simulink subsystem "Day1_Scenario_2"  (R2024a)
settings: Solver=VariableStepAuto  StartTime=0.0  StopTime=10.0  RelTol=1e-3
libraries: CarMaker4SL x2
settings Model: Creator=junhyung.cha  LastModifiedBy=User

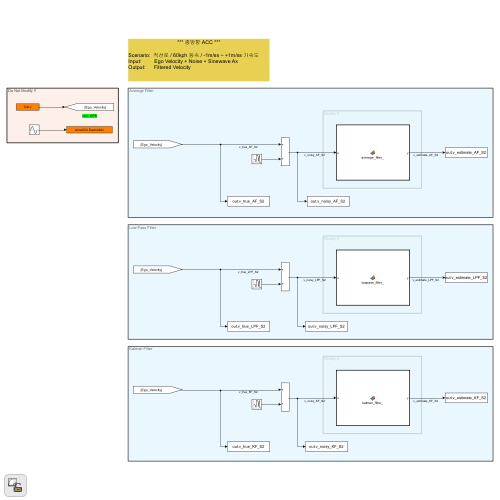
[thumbnail: Simulink's stored preview of the top-level diagram]
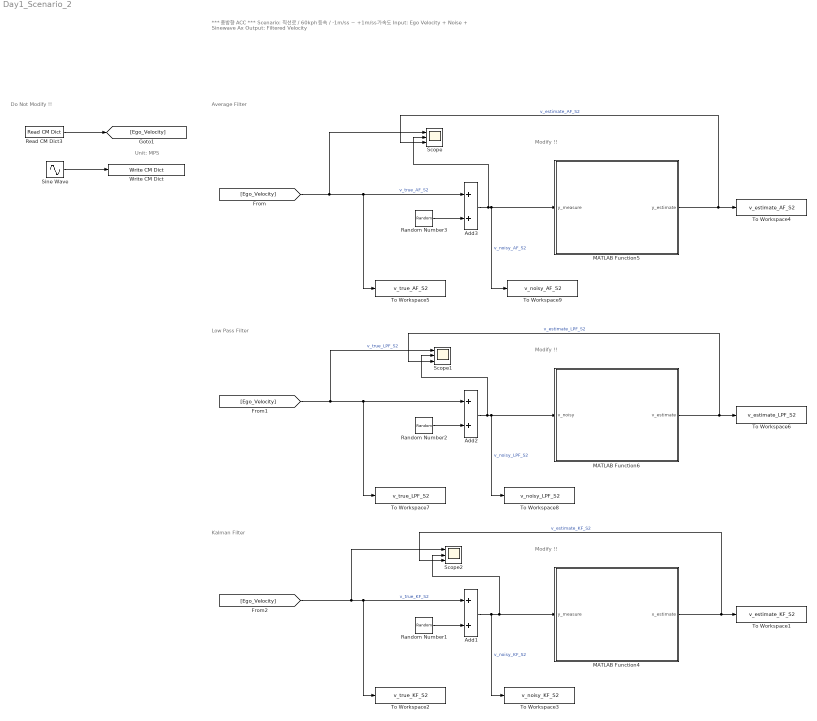
== system Day1_Scenario_2 ==
  note: Do Not Modify !!
  note: Low Pass Filter
  note: Average Filter
  note: Modify !!
  note: Modify !!
  note: Kalman Filter
  note: Modify !!
  note: *** 종방향 ACC ***
      |
      | Scenario: 직선로 / 60kph 등속 / -1m/ss ~ +1m/ss 가속도
      | Input: Ego Velocity + Noise + Sinewave Ax
      | Output: Filtered Velocity
  note: Unit: MPS
  Add1 : Sum
  Add2 : Sum
  Add3 : Sum
  MATLAB Function4 : MATLAB Function  TreatAsAtomicUnit=on
  MATLAB Function5 : MATLAB Function  TreatAsAtomicUnit=on
  MATLAB Function6 : MATLAB Function  TreatAsAtomicUnit=on
  Random Number1 : RandomNumber
  Random Number2 : RandomNumber
  Random Number3 : RandomNumber
  Read CM Dict3 : CarMaker4SL/Read CM Dict  xname=Car.v  xsync=off  xstime=Inherited
  Scope : Scope  NumInputPorts=3
  Scope1 : Scope  NumInputPorts=3
  Scope2 : Scope  NumInputPorts=3
  Sine Wave : Sin
  To Workspace1 : ToWorkspace  VariableName=v_estimate_KF_S2  SaveFormat=Timeseries  SampleTime=-1
  To Workspace2 : ToWorkspace  VariableName=v_true_KF_S2  SaveFormat=Timeseries  SampleTime=-1
  To Workspace3 : ToWorkspace  VariableName=v_noisy_KF_S2  SaveFormat=Timeseries  SampleTime=-1
  To Workspace4 : ToWorkspace  VariableName=v_estimate_AF_S2  SaveFormat=Timeseries  SampleTime=-1
  To Workspace5 : ToWorkspace  VariableName=v_true_AF_S2  SaveFormat=Timeseries  SampleTime=-1
  To Workspace6 : ToWorkspace  VariableName=v_estimate_LPF_S2  SaveFormat=Timeseries  SampleTime=-1
  To Workspace7 : ToWorkspace  VariableName=v_true_LPF_S2  SaveFormat=Timeseries  SampleTime=-1
  To Workspace8 : ToWorkspace  VariableName=v_noisy_LPF_S2  SaveFormat=Timeseries  SampleTime=-1
  To Workspace9 : ToWorkspace  VariableName=v_noisy_AF_S2  SaveFormat=Timeseries  SampleTime=-1
  Write CM Dict : CarMaker4SL/Write CM Dict  xname=AccelCtrl.DesiredAx  xsync=off
  wires:
  Sine Wave/1 -> Write CM Dict/1
  Random Number3/1 -> Add3/2
  Add3/1 -> To Workspace9/1, MATLAB Function5/1(y_measure), Scope/2  "v_noisy_AF_S2"
  Add2/1 -> To Workspace8/1, MATLAB Function6/1(v_noisy), Scope1/2  "v_noisy_LPF_S2"
  [Ego_Velocity] -> Add2/1, To Workspace7/1, Scope1/1  "v_true_LPF_S2"
  MATLAB Function6/1(v_estimate) -> To Workspace6/1, Scope1/3  "v_estimate_LPF_S2"
  Random Number2/1 -> Add2/2
  MATLAB Function5/1(y_estimate) -> To Workspace4/1, Scope/3  "v_estimate_AF_S2"
  Add1/1 -> To Workspace3/1, MATLAB Function4/1(y_measure), Scope2/2  "v_noisy_KF_S2"
  [Ego_Velocity] -> Add1/1, To Workspace2/1, Scope2/1  "v_true_KF_S2"
  MATLAB Function4/1(x_estimate) -> To Workspace1/1, Scope2/3  "v_estimate_KF_S2"
  [Ego_Velocity] -> Add3/1, To Workspace5/1, Scope/1  "v_true_AF_S2"
  Random Number1/1 -> Add1/2
  Read CM Dict3/1 -> [Ego_Velocity]

== matlab function Day1_Scenario_2/MATLAB Function5 ==
  settings: updateMethod=DISCRETE  sampleTime=0.05
  data: y_measure input; y_estimate output
function y_estimate = moving_average_filter_step(y_measure)
% y_measure: 현재 측정값
% y_estimate: 이동 평균 필터 결과

persistent history buffer_idx y_est
n = 17; % 평균 내는 샘플 수 (필요 시 변경 가능)

if isempty(history)
    history = zeros(1, n + 1); % n+1개 저장 (과거 값 추출용)
    history(:) = y_measure;
    buffer_idx = 1;
    y_est = y_measure;
end

% 현재 샘플 저장
buffer_idx = mod(buffer_idx, n + 1) + 1;
history(buffer_idx) = y_measure;

% n+1 샘플 전 값 찾기 (circular buffer)
x_k_n = history(mod(buffer_idx, n + 1) + 1);

% 업데이트
y_est = y_est + (1 / n) * (y_measure - x_k_n);
y_estimate = y_est;

== matlab function Day1_Scenario_2/MATLAB Function6 ==
  settings: updateMethod=DISCRETE  sampleTime=0.05
  data: v_noisy input; v_estimate output
function v_estimate = low_pass_filter_step(v_noisy)
% v_estimate: 필터 출력
% v_noisy: 노이즈가 있는 입력
% 내부 상태 유지 위해 persistent 사용

persistent v_est_prev
alpha = 0.9;

if isempty(v_est_prev)
    v_est_prev = v_noisy;
end

% 필터 식
v_estimate = alpha * v_est_prev + (1 - alpha) * v_noisy;

% 상태 업데이트
v_est_prev = v_estimate;

== matlab function Day1_Scenario_2/MATLAB Function4 ==
  settings: updateMethod=DISCRETE  sampleTime=0.05
  data: y_measure input; x_estimate output
function x_estimate = kalman_filter_step(y_measure)
% y_measure: 현재 측정값 (v_noisy_KF_S1)
% x_estimate: 필터 추정 출력

persistent x_est P_est A B C Q R dt

% 고정된 dt 값 (시간 간격)
if isempty(dt)
    dt = 0.001;  % 샘플링 시간 (예: 0.1초)
end

% 필터 파라미터
if isempty(x_est)
    % 초기화 (필터의 초기 상태 및 공분산)
    A = [1.0, dt; 0.0, 1.0];  % 상태 전이 행렬 (A * dt)
    B = [0.0; dt];             % 입력 제어 행렬 (여기서는 입력 없음)
    C = [1.0, 0.0];            % 측정 행렬
    Q = [0.01, 0; 0, 0.01];    % 모델 노이즈 공분산
    R = 1.0;                   % 측정 노이즈 공분산
    x_est = [y_measure; 0.0];  % 초기 상태 추정 (위치, 속도)
    P_est = [10.0, 0.0; 0.0, 10.0];  % 초기 공분산
end

% Prediction (예측)
A_dt = A * dt + eye(size(A));  % 상태 전이 행렬 업데이트 (Adt + I)
x_pred = A_dt * x_est;         % 예측된 상태
P_pred = A_dt * P_est * A_dt' + Q;  % 공분산 예측

% Kalman Gain 계산
S = C * P_pred * C' + R;  % S 계산
K = P_pred * C' / S;      % 칼만 이득 계산

% Update (업데이트)
y_error = y_measure - C * x_pred;  % 측정 오차
x_est = x_pred + K * y_error;      % 상태 추정 업데이트
P_est = (eye(size(P_est)) - K * C) * P_pred;  % 공분산 업데이트

% 출력
x_estimate = x_est;  % 최종 상태 추정값 출력
end
